simulink model "CS_SUP"  (Simulink 8.7)
settings: Solver=ode45  StartTime=0.0  StopTime=inf  RelTol=1e-3
values from neighbouring files (symbols this model uses):
  Ex = 10^(0.1*SNR_Current)    [main.m]
  Frame_Len = 512    [Walsh.m]    (also in main.m)
  K = K_ChannelDim    (= 32)    [main.m]
  K_ChannelDim = 32    [main.m]
  pho = 0.05    [main.m]
  Sample_time = 1    [main.m]
undefined symbols (not defined in the file or in its folder): magnitude
libraries: commdigbbndpm3 x2, commrandsrc2 x1, commsink2 x1, dspstat3 x1
settings Model: Creator=QCJ  LastModifiedBy=杜红
settings DataIOCC: SignalLoggingSaveFormat=ModelDataLogs  InspectSignalLogs=on
settings OptimizationCC: InitFltsAndDblsToZero=on
settings DebuggingCC: SaveWithParameterizedLinksMsg=none  SignalResolutionControl=TryResolveAllWithWarning  SolverPrmCheckMsg=warning  MultiTaskDSMMsg=warning  MultiTaskCondExecSysMsg=none  FcnCallInpInsideContextMsg=UseLocalSettings
settings GRTTargetCC: TargetFcnLib=ansi_tfl_tmw.mat  CombineOutputUpdateFcns=off  GRTInterface=on
settings ConfigComp: CovSFcnEnable=off

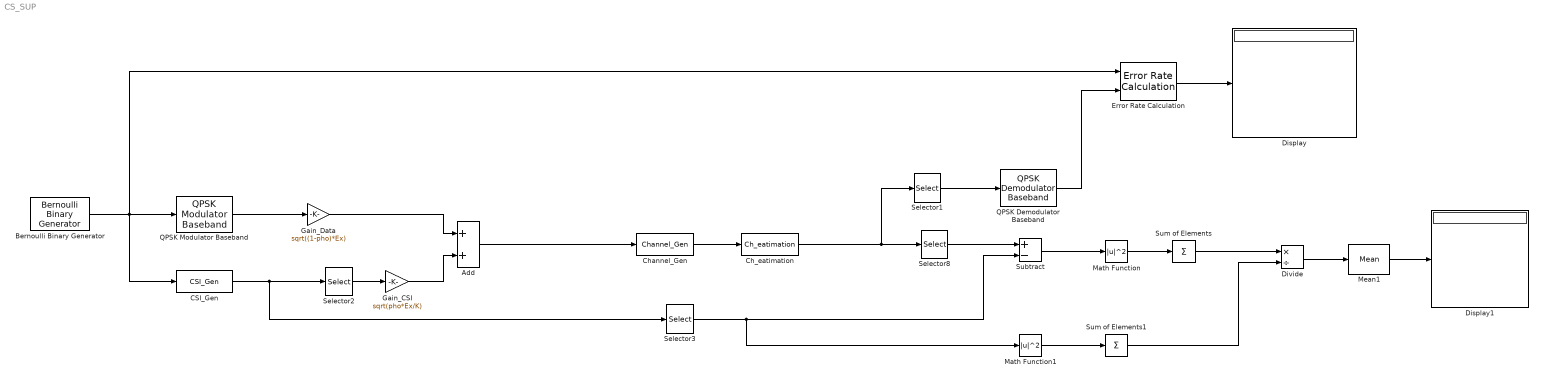
== system CS_SUP ==
  Add : Sum
  Bernoulli Binary Generator : commrandsrc2/Bernoulli Binary Generator  P=0.5  seed=61  Ts=Sample_time  frameBased=on  sampPerFrame=Frame_Len*2  orient=off  outDataType=double
  CSI_Gen : MATLABFcn  MATLABFcn=CSI_Gen  OutputSignalType=complex  Output1D=off
  Ch_eatimation : MATLABFcn  MATLABFcn=Ch_eatimation  OutputSignalType=complex  Output1D=off
  Channel_Gen : MATLABFcn  MATLABFcn=Channel_Gen  OutputSignalType=complex  Output1D=off
  Display : Display
  Display1 : Display
  Divide : Product  Inputs=*/
  Error Rate Calculation : commsink2/Error Rate Calculation  N=0  st_delay=0  cp_mode=Entire frame  subframe=[]  PMode=Port  WsName=ErrorVec  RsMode2=off  stop=off  numErr=100  maxBits=1e6
  Gain_CSI : Gain  Gain=sqrt(pho*Ex/K)
  Gain_Data : Gain  Gain=sqrt((1-pho)*Ex)
  Math Function : Math  Operator=magnitude^2  SaturateOnIntegerOverflow=on
  Math Function1 : Math  Operator=magnitude^2  SaturateOnIntegerOverflow=on
  Mean1 : dspstat3/Mean  run=on  reset_popup=None  InputProcessing=Columns as channels (frame based)  directionMode=Entire input  dimension=1  roiEnable=off  roiType=Rectangles  roiPortion=Entire ROI  roiOutput=Individual statistics for each ROI  roiFlag=off  outputDataTypeStr=Inherit: Same as accumulator  outputLastDataTypeStr=Inherit: Same as accumulator  outputMin=[]  outputMax=[]  roundingMode=Floor  overflowMode=off
  QPSK Demodulator Baseband : commdigbbndpm3/QPSK Demodulator Baseband  OutType=Bit  DecType=Hard decision  VarSource=Dialog  Variance=1  Dec=Gray  Ph=pi/4  outDtype1=Inherit via internal rule  outDtype2=Inherit via internal rule  derotateFactorWordLen=16  derotateFactorDataTypeStr=Inherit: Same word length as input  derotateFactorLastDataTypeStr=Inherit: Same word length as input
  QPSK Modulator Baseband : commdigbbndpm3/QPSK Modulator Baseband  InType=Bit  Enc=Gray  Ph=pi/4  outDtype=double  outWordLen=16  outUDDataType=sfix(16)  outFracLenMode=Best precision  outFracLen=15  outDataTypeStr=double  outLastDataTypeStr=double
  Selector1 : Selector  InputPortWidth=K_ChannelDim + Frame_Len  IndexOptions=Index vector (dialog)  Indices=[K_ChannelDim+1:K_ChannelDim + Frame_Len]  OutputSizes=1
  Selector2 : Selector  InputPortWidth=K_ChannelDim + Frame_Len  IndexOptions=Index vector (dialog)  Indices=[K_ChannelDim+1:K_ChannelDim + Frame_Len]  OutputSizes=1
  Selector3 : Selector  InputPortWidth=K_ChannelDim + Frame_Len  IndexOptions=Index vector (dialog)  Indices=[1:K_ChannelDim]  OutputSizes=1
  Selector8 : Selector  InputPortWidth=K_ChannelDim + Frame_Len  IndexOptions=Index vector (dialog)  Indices=[1:K_ChannelDim]  OutputSizes=1
  Subtract : Sum  Inputs=+-
  Sum of Elements : Sum  Inputs=+
  Sum of Elements1 : Sum  Inputs=+
  wires:
  QPSK Modulator Baseband/1 -> Gain_Data/1
  Gain_Data/1 -> Add/1
  CSI_Gen/1 -> Selector2/1, Selector3/1
  Gain_CSI/1 -> Add/2
  Channel_Gen/1 -> Ch_eatimation/1
  Ch_eatimation/1 -> Selector1/1, Selector8/1
  Selector8/1 -> Subtract/1
  Selector1/1 -> QPSK Demodulator Baseband/1
  Selector2/1 -> Gain_CSI/1
  Selector3/1 -> Math Function1/1, Subtract/2
  QPSK Demodulator Baseband/1 -> Error Rate Calculation/2
  Error Rate Calculation/1 -> Display/1
  Bernoulli Binary Generator/1 -> Error Rate Calculation/1, CSI_Gen/1, QPSK Modulator Baseband/1
  Subtract/1 -> Math Function/1
  Math Function/1 -> Sum of Elements/1
  Math Function1/1 -> Sum of Elements1/1
  Sum of Elements1/1 -> Divide/2
  Mean1/1 -> Display1/1
  Sum of Elements/1 -> Divide/1
  Divide/1 -> Mean1/1
  Add/1 -> Channel_Gen/1
